simulink model "Continuity_PDE_ConservationTest"  (R2019a)
settings: Solver=VariableStepAuto  StartTime=0.0  StopTime=13  FixedStep=0.01  MaxStep=0.01  RelTol=1e-3
libraries: PDECharactLib x1
settings Model: Creator=kc5492  LastModifiedBy=kc5492
settings SolverCC: ZeroCrossAlgorithm=Adaptive
settings DataIOCC: ReturnWorkspaceOutputs=off
settings DebuggingCC: PregeneratedLibrarySubsystemCodeDiagnostic=none  ArithmeticOperatorsInVariantConditions=warning
settings SFSimCC: SimUseLocalCustomCode=off
settings RTWCC: RTWUseLocalCustomCode=off

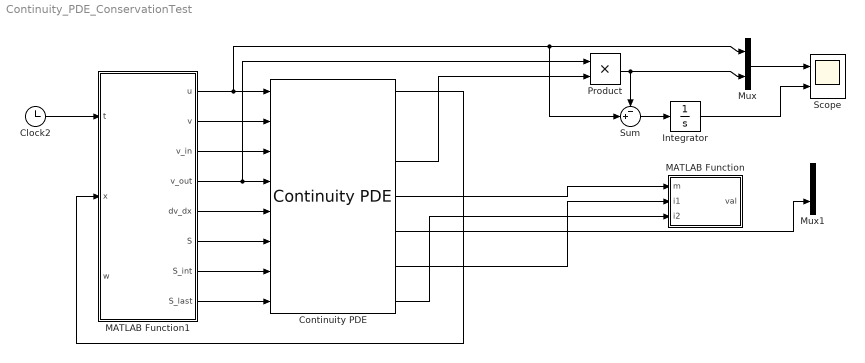
== system Continuity_PDE_ConservationTest ==
  Clock2 : Clock
  Continuity PDE : PDECharactLib/Continuity PDE  ell=1  Nmax=100  x0=0:0.1:1  w0=zeros(1,11)  m0=zeros(1,10)  initM_tot=0  initX=0  initW=0  initM=0  dx=0.1  dw=inf  dt=0.1  crossing_tol=1e-11  overflow_err=off
  Integrator : Integrator
  MATLAB Function : MATLAB Function  TreatAsAtomicUnit=on
  MATLAB Function1 : MATLAB Function  TreatAsAtomicUnit=on
  Mux : Mux  Inputs=2
  Mux1 : Mux  Inputs=2
  Product : Product
  Scope : Scope  NumInputPorts=2
  Sum : Sum  Inputs=-+|
  wires:
  Clock2/1 -> MATLAB Function1/1(t)
  Sum/1 -> Integrator/1
  MATLAB Function1/1(u) -> Sum/2, Mux/1, Continuity PDE/1
  Continuity PDE/1 -> MATLAB Function1/2(x)
  MATLAB Function1/2(v) -> Continuity PDE/2
  MATLAB Function1/5(dv_dx) -> Continuity PDE/5
  MATLAB Function1/6(S) -> Continuity PDE/6
  MATLAB Function1/7(S_int) -> Continuity PDE/7
  MATLAB Function1/8(S_last) -> Continuity PDE/8
  Product/1 -> Sum/1, Mux/2
  Mux/1 -> Scope/1
  MATLAB Function1/4(v_out) -> Product/1, Continuity PDE/4
  Continuity PDE/3 -> Product/2
  MATLAB Function1/3(v_in) -> Continuity PDE/3
  Continuity PDE/4 -> MATLAB Function/1(m)
  Continuity PDE/6 -> MATLAB Function/2(i1)
  Continuity PDE/7 -> MATLAB Function/3(i2)
  Continuity PDE/5 -> Mux1/2
  Integrator/1 -> Scope/2

== matlab function Continuity_PDE_ConservationTest/MATLAB Function1 ==
  data: u output; t input; v output; v_in output; x input; w input; v_out output; dv_dx output; S output; S_int output; S_last output
function [u, v, v_in, v_out, dv_dx, S, S_int, S_last] = equationTerms(t, x, w)

% ell = 1

v = x + 1.1 + sin(t);
v_in = 0 + 1.1 + sin(t);
v_out = 1 + 1.1 + sin(t);
dv_dx = ones(length(x), 1);
S = 0*x;
S_int = 0*x;
S_last = 0;
u = (t >= 2) * (t <= 10) * (1 + cos(pi/2*t))/2;

== matlab function Continuity_PDE_ConservationTest/MATLAB Function ==
  data: m input; i1 input; val output; i2 input
function val = tester(m, i1, i2)

if i1 < i2
    ind = i1:i2;
else
    ind = [i1:100, 1:i2];
end

val = length(ind);
